simulink subsystem "component_level_execution"  (R2022b)
settings: Solver=VariableStepAuto  StartTime=0.0  StopTime=10.0  RelTol=1e-3
settings Model: Creator=micha  LastModifiedBy=micha
settings ModelReferenceCC: EnableRefExpFcnMdlSchedulingChecks=on

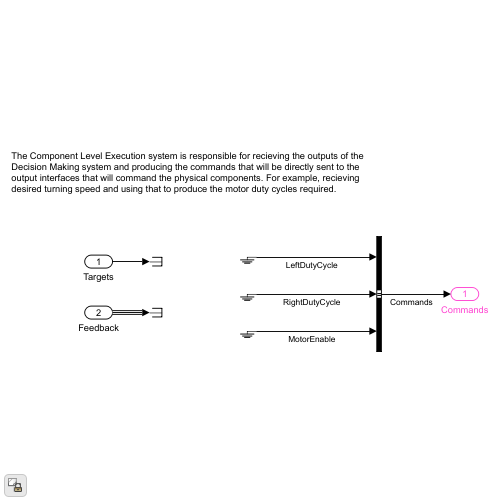
[thumbnail: Simulink's stored preview of the top-level diagram]
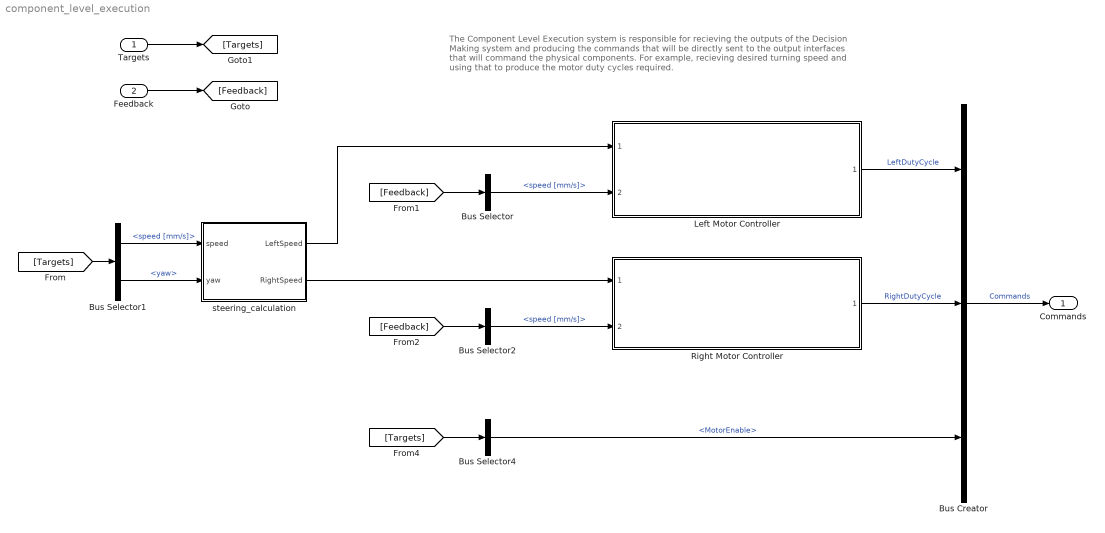
== system component_level_execution ==
  note: The Component Level Execution system is responsible for recieving the outputs of the Decision Making system and producing the commands that will be directly sent to the output interfaces that will command the physical components. For example, recieving desired turning speed and using that to produce the motor duty cycles required.
  Targets : Inport
  Feedback : Inport  Port=2
  Bus Creator : BusCreator  Inputs=3
  Bus Selector : BusSelector  OutputSignals=LeftWheel.speed [mm/s]
  Bus Selector1 : BusSelector  OutputSignals=speed [mm/s],yaw
  Bus Selector2 : BusSelector  OutputSignals=RightWheel.speed [mm/s]
  Bus Selector4 : BusSelector  OutputSignals=MotorEnable
  Left Motor Controller : Subsystem  ReferencedSubsystem=motor_controller
  Right Motor Controller : Subsystem  ReferencedSubsystem=motor_controller
  steering_calculation : Subsystem
  Commands : Outport
  wires:
  Targets/1 -> [Targets]
  Feedback/1 -> [Feedback]
  Left Motor Controller/1 -> Bus Creator/1  "LeftDutyCycle"
  Right Motor Controller/1 -> Bus Creator/2  "RightDutyCycle"
  Bus Selector4/1 -> Bus Creator/3  "<MotorEnable>"
  Bus Creator/1 -> Commands/1  "Commands"
  [Feedback] -> Bus Selector/1
  Bus Selector/1 -> Left Motor Controller/2  "<speed [mm/s]>"
  [Targets] -> Bus Selector1/1
  Bus Selector1/1 -> steering_calculation/1(speed)  "<speed [mm/s]>"
  Bus Selector2/1 -> Right Motor Controller/2  "<speed [mm/s]>"
  [Feedback] -> Bus Selector2/1
  [Targets] -> Bus Selector4/1
  Bus Selector1/2 -> steering_calculation/2(yaw)  "<yaw>"
  steering_calculation/1(LeftSpeed) -> Left Motor Controller/1
  steering_calculation/2(RightSpeed) -> Right Motor Controller/1

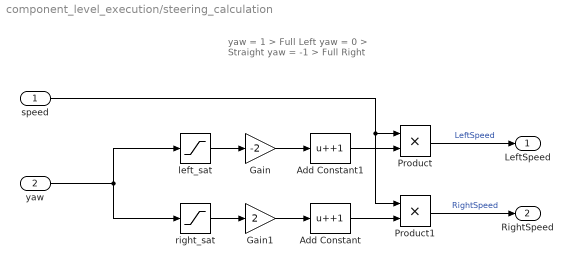
== system component_level_execution/steering_calculation ==
  note: yaw = 1   >  Full Left
      | yaw = 0   >  Straight
      | yaw = -1  >  Full Right
  speed : Inport
  yaw : Inport  Port=2
  Add Constant : Bias  Bias=+1  SaturateOnIntegerOverflow=off
  Add Constant1 : Bias  Bias=+1  SaturateOnIntegerOverflow=off
  Gain : Gain  Gain=-2
  Gain1 : Gain  Gain=2
  Product : Product
  Product1 : Product
  left_sat : Saturate  UpperLimit=1  LowerLimit=0
  right_sat : Saturate  UpperLimit=0  LowerLimit=-1
  LeftSpeed : Outport
  RightSpeed : Outport  Port=2
  wires:
  Product1/1 -> RightSpeed/1  "RightSpeed"
  Product/1 -> LeftSpeed/1  "LeftSpeed"
  Add Constant/1 -> Product1/2
  Add Constant1/1 -> Product/2
  Gain/1 -> Add Constant1/1
  Gain1/1 -> Add Constant/1
  right_sat/1 -> Gain1/1
  left_sat/1 -> Gain/1
  yaw/1 -> right_sat/1, left_sat/1
  speed/1 -> Product/1, Product1/1
